simulink model "RCAM_sim"  (R2023a)
settings: Solver=VariableStepAuto  StartTime=0.0  StopTime=t_sim  RelTol=1e-3
InitFcn:
  | % clc
  | % clear
  | % RCAM_init
  | % RCAM_init_trimmed
  | RCAM_constants
  | 
  | % Independent run (Untrimmed): Use lines 1,2,3,5
  | % Independent run (Trimmed): Use lines 1,2,4,5
  | % Trimming: Use line 5 only
values from neighbouring files (symbols this model uses):
  a0 = 15.212    [RCAM0_model.m]    (also in RCAM_constants.m; RCAM_constants.mat)
  a1 = -155.2    [RCAM0_model.m]    (also in RCAM_constants.m; RCAM_constants.mat)
  a2 = 609.2    [RCAM0_model.m]    (also in RCAM_constants.m; RCAM_constants.mat)
  a3 = -768.5    [RCAM0_model.m]    (also in RCAM_constants.m; RCAM_constants.mat)
  alpha_L0 = deg2rad(-11.5)    [RCAM0_model.m]    (also in RCAM_constants.m; RCAM_constants.mat = -0.200712863979)
  alpha_switch = deg2rad(14.5)    [RCAM0_model.m]    (also in RCAM_constants.m; RCAM_constants.mat = 0.253072741539)
  cbar = 6.6    [RCAM0_model.m]    (also in RCAM_constants.m; RCAM_constants.mat)
  cd_c1 = 0.654    [RCAM_constants.m]    (also in RCAM_constants.mat)
  cd_c2 = 0.13    [RCAM_constants.m]    (also in RCAM_constants.mat)
  cd_m1 = 5.5    [RCAM_constants.m]    (also in RCAM_constants.mat)
  cd_m2 = 0.07    [RCAM_constants.m]    (also in RCAM_constants.mat)
  dCYdbeta = -1.6    [RCAM_constants.m]    (also in RCAM_constants.mat)
  dCYdRud = 0.24    [RCAM_constants.m]    (also in RCAM_constants.mat)
  depsda = 0.25    [RCAM0_model.m]    (also in RCAM_constants.m; RCAM_constants.mat)
  dumax = deg2rad(dumax)    [RCAM_constants.m]    (also in RCAM_constants.mat = [1.0471975512 1.0471975512 1.0471975512 0.0349065850399 0.03)
  g = 9.81    [RCAM0_model.m]    (also in RCAM_constants.m; RCAM_constants.mat)
  lt = 24.8    [RCAM0_model.m]    (also in RCAM_constants.m; RCAM_constants.mat)
  m = 120000    [RCAM0_model.m]    (also in RCAM_constants.m; RCAM_constants.mat)
  n = 5.5    [RCAM0_model.m]    (also in RCAM_constants.m; RCAM_constants.mat)
  S = 260    [RCAM0_model.m]    (also in RCAM_constants.m; RCAM_constants.mat)
  St = 64    [RCAM0_model.m]    (also in RCAM_constants.m; RCAM_constants.mat)
  u0 = [0 ... (first row only)    [RCAM0_init.m]    (also in RCAM_constants.mat = [0 -0.194874130949 0 0.0795600512836 0.0795600512836]; RCAM_dynamics.m = u; RCAM_init.m = deg2rad(u0); RCAM_init2.m = ustar)
  umax = deg2rad(umax)    [RCAM0_model.m]    (also in RCAM_constants.m; RCAM_constants.mat = [0.436332312999 0.174532925199 0.523598775598 0.174532925199)
  umin = deg2rad(umin)    [RCAM0_model.m]    (also in RCAM_constants.m; RCAM_constants.mat = [-0.436332312999 -0.436332312999 -0.523598775598 0.008726646)
  Xac = 0.12*cbar    (= 0.792)    [RCAM0_model.m]    (also in RCAM_constants.m; RCAM_constants.mat)
  Xcg = 0.23*cbar    (= 1.518)    [RCAM0_model.m]    (also in RCAM_constants.m; RCAM_constants.mat)
  Yac = 0    [RCAM0_model.m]    (also in RCAM_constants.m; RCAM_constants.mat)
  Ycg = 0    [RCAM0_model.m]    (also in RCAM_constants.m; RCAM_constants.mat)
  Zac = 0    [RCAM0_model.m]    (also in RCAM_constants.m; RCAM_constants.mat)
  Zcg = 0.1*cbar    (= 0.66)    [RCAM0_model.m]    (also in RCAM_constants.m; RCAM_constants.mat)
libraries: simulink_extras x12, aerolibactuator x5, slpidlib x3, matrix_library x3, sharedutil x2, shared6dof x1, aerolibatmos2 x1
settings Model: Creator=Reggie Johanes  LastModifiedBy=Reggie Johanes

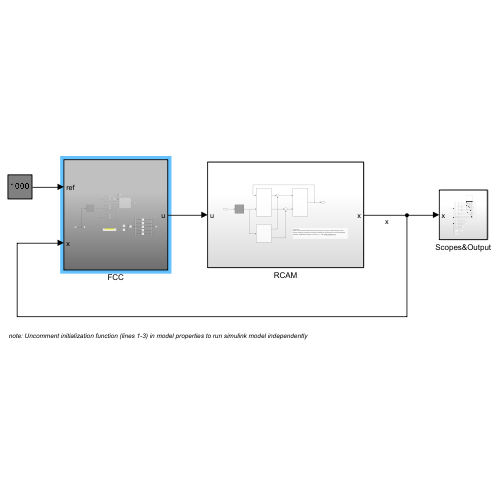
[thumbnail: Simulink's stored preview of the top-level diagram]
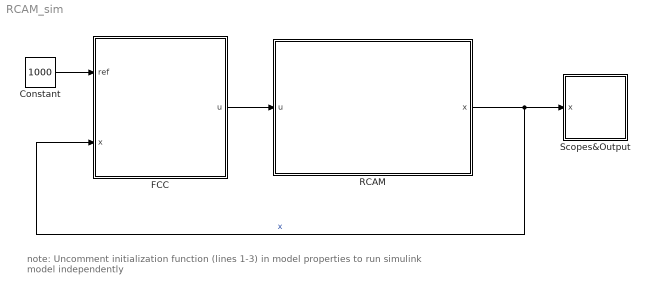
== system RCAM_sim ==
  note: note: Uncomment initialization function (lines 1-3) in model properties to run simulink model independently
  Constant : Constant  Value=1000
  FCC : Subsystem
  RCAM : Subsystem
  Scopes&Output : Subsystem
  wires:
  FCC/1(u) -> RCAM/1(u)
  RCAM/1(x) -> FCC/2(x), Scopes&Output/1(x)  "x"
  Constant/1 -> FCC/1(ref)

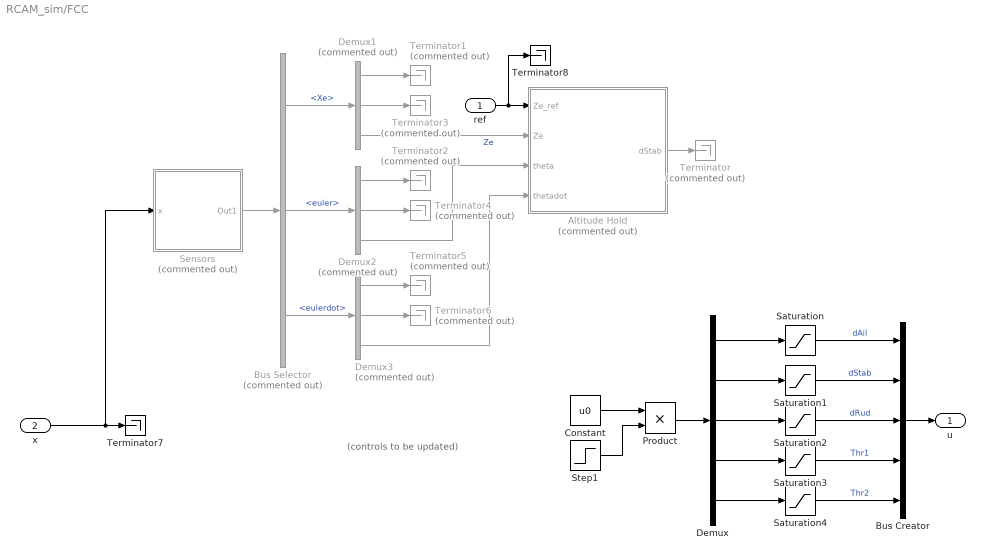
== system RCAM_sim/FCC ==
  note: (controls to be updated)
  ref : Inport
  x : Inport  Port=2
  Altitude Hold : Subsystem  Commented=on
  Bus Creator : BusCreator  Inputs=5
  Bus Selector : BusSelector  Commented=on  OutputSignals=Xe,euler,eulerdot
  Constant : Constant  Value=u0
  Demux : Demux  Outputs=5
  Demux1 : Demux  Commented=on  Outputs=3
  Demux2 : Demux  Commented=on  Outputs=3
  Demux3 : Demux  Commented=on  Outputs=3
  Product : Product
  Saturation : Saturate  UpperLimit=umax(1)  LowerLimit=umin(1)
  Saturation1 : Saturate  UpperLimit=umax(2)  LowerLimit=umin(2)
  Saturation2 : Saturate  UpperLimit=umax(3)  LowerLimit=umin(3)
  Saturation3 : Saturate  UpperLimit=umax(4)  LowerLimit=umin(4)
  Saturation4 : Saturate  UpperLimit=umax(5)  LowerLimit=umin(5)
  Sensors : Subsystem  Commented=on
  Step1 : Step  Time=0  SampleTime=0
  Terminator{,1..6} (7 alike) : Terminator  Commented=on
  Terminator7 : Terminator
  Terminator8 : Terminator
  u : Outport
  wires:
  ref/1 -> Terminator8/1, Altitude Hold/1(Ze_ref)
  x/1 -> Sensors/1(x), Terminator7/1
  Step1/1 -> Product/2
  Product/1 -> Demux/1
  Demux/5 -> Saturation4/1
  Demux/4 -> Saturation3/1
  Demux/3 -> Saturation2/1
  Demux/2 -> Saturation1/1
  Demux/1 -> Saturation/1
  Bus Creator/1 -> u/1
  Bus Selector/1 -> Demux1/1  "<Xe>"
  Bus Selector/2 -> Demux2/1  "<euler>"
  Saturation/1 -> Bus Creator/1  "dAil"
  Saturation1/1 -> Bus Creator/2  "dStab"
  Saturation2/1 -> Bus Creator/3  "dRud"
  Saturation3/1 -> Bus Creator/4  "Thr1"
  Saturation4/1 -> Bus Creator/5  "Thr2"
  Demux1/1 -> Terminator1/1
  Demux1/2 -> Terminator3/1
  Bus Selector/3 -> Demux3/1  "<eulerdot>"
  Demux1/3 -> Altitude Hold/2(Ze)  "Ze"
  Demux2/2 -> Terminator4/1
  Demux2/1 -> Terminator2/1
  Demux3/1 -> Terminator5/1
  Demux3/2 -> Terminator6/1
  Demux2/3 -> Altitude Hold/3(theta)
  Demux3/3 -> Altitude Hold/4(thetadot)
  Constant/1 -> Product/1
  Altitude Hold/1(dStab) -> Terminator/1
  Sensors/1(Out1) -> Bus Selector/1

== system RCAM_sim/RCAM ==
  note: Reference:
      | Group for Aeronautical Research and Technology in Europe, "Robust Flight Control Design Challenge Problem Formulation and Manual: the Research Civil Aircraft Model (RCAM)", GARTEUR/TP-0883. February 17, 1997 ( https://garteur.org )
  u : Inport
  Actuators : Subsystem
  Aerodynamics : Subsystem
  EOM&Environment : Subsystem
  Propulsion : Subsystem
  Sum : Sum  Inputs=|++
  Sum1 : Sum  Inputs=|++
  x : Outport
  wires:
  u/1 -> Actuators/1(In1)
  Aerodynamics/1(F_a) -> Sum/1
  Aerodynamics/2(M_a) -> Sum1/1
  Sum/1 -> EOM&Environment/1(F)
  Sum1/1 -> EOM&Environment/2(M)
  Propulsion/1(F_e) -> Sum/2
  Propulsion/2(M_e) -> Sum1/2
  EOM&Environment/1(x) -> Aerodynamics/1(x), x/1
  Actuators/1(Out1) -> Propulsion/1(u), Aerodynamics/2(u)

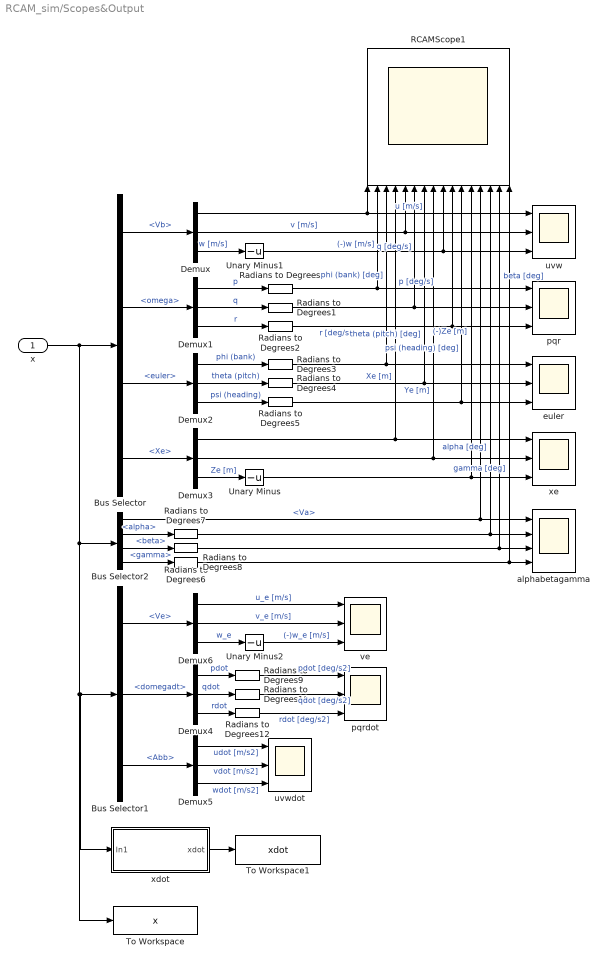
== system RCAM_sim/Scopes&Output ==
  x : Inport
  Bus Selector : BusSelector  OutputSignals=Vb,omega,euler,Xe
  Bus Selector1 : BusSelector  OutputSignals=Ve,domegadt,Abb
  Bus Selector2 : BusSelector  OutputSignals=Va,alpha,beta,gamma
  Demux{,1..6} (7 alike) : Demux  Outputs=3
  RCAMScope1 : Scope  NumInputPorts=16
  Radians to Degrees{,1..10,12} (12 alike) : simulink_extras/Transformations/Radians to Degrees
  To Workspace : ToWorkspace  VariableName=x  SaveFormat=Timeseries  SampleTime=-1
  To Workspace1 : ToWorkspace  VariableName=xdot  SampleTime=-1
  Unary Minus : UnaryMinus
  Unary Minus1 : UnaryMinus
  Unary Minus2 : UnaryMinus
  alphabetagamma : Scope  NumInputPorts=4
  euler : Scope  NumInputPorts=3
  pqr : Scope  NumInputPorts=3
  pqrdot : Scope  NumInputPorts=3
  uvw : Scope  NumInputPorts=3
  uvwdot : Scope  NumInputPorts=3
  ve : Scope  NumInputPorts=3
  xdot : Subsystem
  xe : Scope  NumInputPorts=3
  wires:
  x/1 -> To Workspace/1, xdot/1(In1), Bus Selector1/1, Bus Selector2/1, Bus Selector/1
  Bus Selector/1 -> Demux/1  "<Vb>"
  Bus Selector/2 -> Demux1/1  "<omega>"
  Bus Selector/3 -> Demux2/1  "<euler>"
  Demux/1 -> uvw/1, RCAMScope1/1  "u [m/s]"
  Demux1/2 -> Radians to Degrees1/1  "q"
  Demux/3 -> Unary Minus1/1  "w [m/s]"
  Demux/2 -> uvw/2, RCAMScope1/5  "v [m/s]"
  Demux1/1 -> Radians to Degrees/1  "p"
  Demux1/3 -> Radians to Degrees2/1  "r"
  Demux2/2 -> Radians to Degrees4/1  "theta (pitch)"
  Demux2/3 -> Radians to Degrees5/1  "psi (heading)"
  Bus Selector/4 -> Demux3/1  "<Xe>"
  Demux3/1 -> xe/1, RCAMScope1/4  "Xe [m]"
  Demux3/2 -> xe/2, RCAMScope1/8  "Ye [m]"
  Demux3/3 -> Unary Minus/1  "Ze [m]"
  Demux2/1 -> Radians to Degrees3/1  "phi (bank)"
  Demux4/3 -> Radians to Degrees12/1  "rdot"
  Demux4/2 -> Radians to Degrees10/1  "qdot"
  Bus Selector1/2 -> Demux4/1  "<domegadt>"
  Demux4/1 -> Radians to Degrees9/1  "pdot"
  Demux5/1 -> uvwdot/1  "udot [m/s2]"
  Bus Selector1/3 -> Demux5/1  "<Abb>"
  Demux5/2 -> uvwdot/2  "vdot [m/s2]"
  Demux5/3 -> uvwdot/3  "wdot [m/s2]"
  Radians to Degrees/1 -> pqr/1, RCAMScope1/2  "p [deg/s]"
  Radians to Degrees1/1 -> pqr/2, RCAMScope1/6  "q [deg/s]"
  Radians to Degrees2/1 -> pqr/3, RCAMScope1/10  "r [deg/s]"
  Radians to Degrees3/1 -> euler/1, RCAMScope1/3  "phi (bank) [deg]"
  Radians to Degrees4/1 -> euler/2, RCAMScope1/7  "theta (pitch) [deg]"
  Radians to Degrees5/1 -> euler/3, RCAMScope1/11  "psi (heading) [deg]"
  Unary Minus/1 -> xe/3, RCAMScope1/12  "(-)Ze [m]"
  Bus Selector2/3 -> Radians to Degrees6/1  "<beta>"
  Bus Selector2/1 -> RCAMScope1/13, alphabetagamma/1  "<Va>"
  Bus Selector2/2 -> Radians to Degrees7/1  "<alpha>"
  Radians to Degrees6/1 -> RCAMScope1/15, alphabetagamma/3  "beta [deg]"
  Radians to Degrees7/1 -> RCAMScope1/14, alphabetagamma/2  "alpha [deg]"
  Demux6/3 -> Unary Minus2/1  "w_e"
  Demux6/2 -> ve/2  "v_e [m/s]"
  Bus Selector1/1 -> Demux6/1  "<Ve>"
  Demux6/1 -> ve/1  "u_e [m/s]"
  Unary Minus2/1 -> ve/3  "(-)w_e [m/s]"
  Unary Minus1/1 -> uvw/3, RCAMScope1/9  "(-)w [m/s]"
  Bus Selector2/4 -> Radians to Degrees8/1  "<gamma>"
  Radians to Degrees8/1 -> RCAMScope1/16, alphabetagamma/4  "gamma [deg]"
  Radians to Degrees9/1 -> pqrdot/1  "pdot [deg/s2]"
  Radians to Degrees10/1 -> pqrdot/2  "qdot [deg/s2]"
  Radians to Degrees12/1 -> pqrdot/3  "rdot [deg/s2]"
  xdot/1(xdot) -> To Workspace1/1

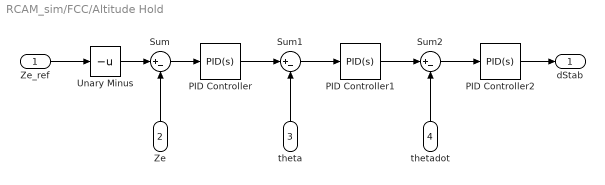
== system RCAM_sim/FCC/Altitude Hold ==
  Ze_ref : Inport
  Ze : Inport  Port=2
  theta : Inport  Port=3
  thetadot : Inport  Port=4
  PID Controller : slpidlib/PID Controller  Controller=PID  Form=Parallel  TimeDomain=Continuous-time  UseExternalTs=off  SampleTime=-1  IntegratorMethod=Forward Euler  FilterMethod=Forward Euler  ControllerParametersSource=internal  P=-2.5  I=0  UseKiTs=off  D=0  N=100  UseFilter=on  TunerSelectOption=Transfer Function Based (PID Tuner App)  InitialConditionSource=internal  InitialConditionForIntegrator=0  InitialConditionForFilter=0  DifferentiatorICPrevScaledInput=0  ExternalReset=none  TrackingMode=off  Kt=1  LimitOutput=off  SatLimitsSource=internal  UpperSaturationLimit=inf  LowerSaturationLimit=-inf  LinearizeAsGain=on  AntiWindupMode=none  Kb=1  LimitIntegrator=off  UpperIntegratorSaturationLimit=inf  LowerIntegratorSaturationLimit=-inf  POutMin=[]  POutMax=[]  IOutMin=[]  IOutMax=[]  DOutMin=[]  DOutMax=[]  NOutMin=[]  NOutMax=[]  SumOutMin=[]  SumOutMax=[]  SaturationOutMin=[]  SaturationOutMax=[]  PParamMin=[]  PParamMax=[]  IParamMin=[]  IParamMax=[]  DParamMin=[]  DParamMax=[]  NParamMin=[]  NParamMax=[]  KbParamMin=[]  KbParamMax=[]  KtParamMin=[]  KtParamMax=[]  KbOutMin=[]  KbOutMax=[]  KtOutMin=[]  KtOutMax=[]  IntegratorOutMin=[]  IntegratorOutMax=[]  FilterOutMin=[]  FilterOutMax=[]  SumI1OutMin=[]  SumI1OutMax=[]  SumI2OutMin=[]  SumI2OutMax=[]  SumI3OutMin=[]  SumI3OutMax=[]  SumI4OutMin=[]  SumI4OutMax=[]  SumDOutMin=[]  SumDOutMax=[]  DifferentiatorOutMin=[]  DifferentiatorOutMax=[]  FilterDiffOutCoefMin=[]  FilterDiffOutCoefMax=[]  ReciprocalOutMin=[]  ReciprocalOutMax=[]  SumDenOutMin=[]  SumDenOutMax=[]  SumNumOutMin=[]  SumNumOutMax=[]  DivideOutMin=[]  DivideOutMax=[]  UdiffTsProdOutMin=[]  UdiffTsProdOutMax=[]  NTsProdOutMin=[]  NTsProdOutMax=[]  UintegralTsProdOutMin=[]  UintegralTsProdOutMax=[]  UngainTsProdOutMin=[]  UngainTsProdOutMax=[]  ClampingZeroOutDataTypeStr=Inherit: Inherit via back propagation  ClampingZeroOutMin=[]  ClampingZeroOutMax=[]  FilterDenConstantOutDataTypeStr=Inherit: Inherit via back propagation  FilterDenConstantOutMin=[]  FilterDenConstantOutMax=[]  PCopyOutDataTypeStr=Inherit: Inherit via back propagation  PCopyOutMin=[]  PCopyOutMax=[]  NCopyOutDataTypeStr=Inherit: Inherit via back propagation  NCopyOutMin=[]  NCopyOutMax=[]  IntegratorContinuousStateAttributes=''  IntegratorStateMustResolveToSignalObject=off  IntegratorRTWStateStorageClass=Auto  FilterContinuousStateAttributes=''  FilterStateMustResolveToSignalObject=off  FilterRTWStateStorageClass=Auto  ParallelPVariant=InternalParameters  IdealPVariant=Disabled  IVariant=InternalParameters  DVariant=InternalParameters  IntegratorVariant=Continuous  SatVariant=Disabled  AWVariant=Passthrough  PCopyVariant=Disabled  TRVariant=Disabled  FdbkBlocksVariant=Forward  IdealPFdbkVariant=Disabled  SatFdbkVariant=Disabled  DerivativeFilterVariant=ContFilter  NVariant=InternalParameters  NCopyVariant=Disabled  FilterICVariant=InternalICsFilter  IntegratorICVariant=InternalICs  ExternalResetVariant=Disabled  TRSumVariant=Passthrough  SumFdbkVariant=Disabled  SumVariant=Sum_PID  TsampFilterVariant=InternalTs  TsampNgainVariant=Passthrough  TsampIntegralVariant=Disabled_SignalSpec  ExternalSaturationOutDataTypeStr=Inherit: Same as second input
  PID Controller1 : slpidlib/PID Controller  Controller=PID  Form=Parallel  TimeDomain=Continuous-time  UseExternalTs=off  SampleTime=-1  IntegratorMethod=Forward Euler  FilterMethod=Forward Euler  ControllerParametersSource=internal  P=1.5  I=0  UseKiTs=off  D=0  N=100  UseFilter=on  TunerSelectOption=Transfer Function Based (PID Tuner App)  InitialConditionSource=internal  InitialConditionForIntegrator=0  InitialConditionForFilter=0  DifferentiatorICPrevScaledInput=0  ExternalReset=none  TrackingMode=off  Kt=1  LimitOutput=off  SatLimitsSource=internal  UpperSaturationLimit=inf  LowerSaturationLimit=-inf  LinearizeAsGain=on  AntiWindupMode=none  Kb=1  LimitIntegrator=off  UpperIntegratorSaturationLimit=inf  LowerIntegratorSaturationLimit=-inf  POutMin=[]  POutMax=[]  IOutMin=[]  IOutMax=[]  DOutMin=[]  DOutMax=[]  NOutMin=[]  NOutMax=[]  SumOutMin=[]  SumOutMax=[]  SaturationOutMin=[]  SaturationOutMax=[]  PParamMin=[]  PParamMax=[]  IParamMin=[]  IParamMax=[]  DParamMin=[]  DParamMax=[]  NParamMin=[]  NParamMax=[]  KbParamMin=[]  KbParamMax=[]  KtParamMin=[]  KtParamMax=[]  KbOutMin=[]  KbOutMax=[]  KtOutMin=[]  KtOutMax=[]  IntegratorOutMin=[]  IntegratorOutMax=[]  FilterOutMin=[]  FilterOutMax=[]  SumI1OutMin=[]  SumI1OutMax=[]  SumI2OutMin=[]  SumI2OutMax=[]  SumI3OutMin=[]  SumI3OutMax=[]  SumI4OutMin=[]  SumI4OutMax=[]  SumDOutMin=[]  SumDOutMax=[]  DifferentiatorOutMin=[]  DifferentiatorOutMax=[]  FilterDiffOutCoefMin=[]  FilterDiffOutCoefMax=[]  ReciprocalOutMin=[]  ReciprocalOutMax=[]  SumDenOutMin=[]  SumDenOutMax=[]  SumNumOutMin=[]  SumNumOutMax=[]  DivideOutMin=[]  DivideOutMax=[]  UdiffTsProdOutMin=[]  UdiffTsProdOutMax=[]  NTsProdOutMin=[]  NTsProdOutMax=[]  UintegralTsProdOutMin=[]  UintegralTsProdOutMax=[]  UngainTsProdOutMin=[]  UngainTsProdOutMax=[]  ClampingZeroOutDataTypeStr=Inherit: Inherit via back propagation  ClampingZeroOutMin=[]  ClampingZeroOutMax=[]  FilterDenConstantOutDataTypeStr=Inherit: Inherit via back propagation  FilterDenConstantOutMin=[]  FilterDenConstantOutMax=[]  PCopyOutDataTypeStr=Inherit: Inherit via back propagation  PCopyOutMin=[]  PCopyOutMax=[]  NCopyOutDataTypeStr=Inherit: Inherit via back propagation  NCopyOutMin=[]  NCopyOutMax=[]  IntegratorContinuousStateAttributes=''  IntegratorStateMustResolveToSignalObject=off  IntegratorRTWStateStorageClass=Auto  FilterContinuousStateAttributes=''  FilterStateMustResolveToSignalObject=off  FilterRTWStateStorageClass=Auto  ParallelPVariant=InternalParameters  IdealPVariant=Disabled  IVariant=InternalParameters  DVariant=InternalParameters  IntegratorVariant=Continuous  SatVariant=Disabled  AWVariant=Passthrough  PCopyVariant=Disabled  TRVariant=Disabled  FdbkBlocksVariant=Forward  IdealPFdbkVariant=Disabled  SatFdbkVariant=Disabled  DerivativeFilterVariant=ContFilter  NVariant=InternalParameters  NCopyVariant=Disabled  FilterICVariant=InternalICsFilter  IntegratorICVariant=InternalICs  ExternalResetVariant=Disabled  TRSumVariant=Passthrough  SumFdbkVariant=Disabled  SumVariant=Sum_PID  TsampFilterVariant=InternalTs  TsampNgainVariant=Passthrough  TsampIntegralVariant=Disabled_SignalSpec  ExternalSaturationOutDataTypeStr=Inherit: Same as second input
  PID Controller2 : slpidlib/PID Controller  Controller=PID  Form=Parallel  TimeDomain=Continuous-time  UseExternalTs=off  SampleTime=-1  IntegratorMethod=Forward Euler  FilterMethod=Forward Euler  ControllerParametersSource=internal  P=-2.5  I=0  UseKiTs=off  D=0  N=100  UseFilter=on  TunerSelectOption=Transfer Function Based (PID Tuner App)  InitialConditionSource=internal  InitialConditionForIntegrator=0  InitialConditionForFilter=0  DifferentiatorICPrevScaledInput=0  ExternalReset=none  TrackingMode=off  Kt=1  LimitOutput=off  SatLimitsSource=internal  UpperSaturationLimit=inf  LowerSaturationLimit=-inf  LinearizeAsGain=on  AntiWindupMode=none  Kb=1  LimitIntegrator=off  UpperIntegratorSaturationLimit=inf  LowerIntegratorSaturationLimit=-inf  POutMin=[]  POutMax=[]  IOutMin=[]  IOutMax=[]  DOutMin=[]  DOutMax=[]  NOutMin=[]  NOutMax=[]  SumOutMin=[]  SumOutMax=[]  SaturationOutMin=[]  SaturationOutMax=[]  PParamMin=[]  PParamMax=[]  IParamMin=[]  IParamMax=[]  DParamMin=[]  DParamMax=[]  NParamMin=[]  NParamMax=[]  KbParamMin=[]  KbParamMax=[]  KtParamMin=[]  KtParamMax=[]  KbOutMin=[]  KbOutMax=[]  KtOutMin=[]  KtOutMax=[]  IntegratorOutMin=[]  IntegratorOutMax=[]  FilterOutMin=[]  FilterOutMax=[]  SumI1OutMin=[]  SumI1OutMax=[]  SumI2OutMin=[]  SumI2OutMax=[]  SumI3OutMin=[]  SumI3OutMax=[]  SumI4OutMin=[]  SumI4OutMax=[]  SumDOutMin=[]  SumDOutMax=[]  DifferentiatorOutMin=[]  DifferentiatorOutMax=[]  FilterDiffOutCoefMin=[]  FilterDiffOutCoefMax=[]  ReciprocalOutMin=[]  ReciprocalOutMax=[]  SumDenOutMin=[]  SumDenOutMax=[]  SumNumOutMin=[]  SumNumOutMax=[]  DivideOutMin=[]  DivideOutMax=[]  UdiffTsProdOutMin=[]  UdiffTsProdOutMax=[]  NTsProdOutMin=[]  NTsProdOutMax=[]  UintegralTsProdOutMin=[]  UintegralTsProdOutMax=[]  UngainTsProdOutMin=[]  UngainTsProdOutMax=[]  ClampingZeroOutDataTypeStr=Inherit: Inherit via back propagation  ClampingZeroOutMin=[]  ClampingZeroOutMax=[]  FilterDenConstantOutDataTypeStr=Inherit: Inherit via back propagation  FilterDenConstantOutMin=[]  FilterDenConstantOutMax=[]  PCopyOutDataTypeStr=Inherit: Inherit via back propagation  PCopyOutMin=[]  PCopyOutMax=[]  NCopyOutDataTypeStr=Inherit: Inherit via back propagation  NCopyOutMin=[]  NCopyOutMax=[]  IntegratorContinuousStateAttributes=''  IntegratorStateMustResolveToSignalObject=off  IntegratorRTWStateStorageClass=Auto  FilterContinuousStateAttributes=''  FilterStateMustResolveToSignalObject=off  FilterRTWStateStorageClass=Auto  ParallelPVariant=InternalParameters  IdealPVariant=Disabled  IVariant=InternalParameters  DVariant=InternalParameters  IntegratorVariant=Continuous  SatVariant=Disabled  AWVariant=Passthrough  PCopyVariant=Disabled  TRVariant=Disabled  FdbkBlocksVariant=Forward  IdealPFdbkVariant=Disabled  SatFdbkVariant=Disabled  DerivativeFilterVariant=ContFilter  NVariant=InternalParameters  NCopyVariant=Disabled  FilterICVariant=InternalICsFilter  IntegratorICVariant=InternalICs  ExternalResetVariant=Disabled  TRSumVariant=Passthrough  SumFdbkVariant=Disabled  SumVariant=Sum_PID  TsampFilterVariant=InternalTs  TsampNgainVariant=Passthrough  TsampIntegralVariant=Disabled_SignalSpec  ExternalSaturationOutDataTypeStr=Inherit: Same as second input
  Sum : Sum  Inputs=|+-
  Sum1 : Sum  Inputs=|+-
  Sum2 : Sum  Inputs=|+-
  Unary Minus : UnaryMinus
  dStab : Outport
  wires:
  Ze_ref/1 -> Unary Minus/1
  Unary Minus/1 -> Sum/1
  Ze/1 -> Sum/2
  Sum/1 -> PID Controller/1
  Sum1/1 -> PID Controller1/1
  Sum2/1 -> PID Controller2/1
  PID Controller/1 -> Sum1/1
  theta/1 -> Sum1/2
  PID Controller1/1 -> Sum2/1
  thetadot/1 -> Sum2/2
  PID Controller2/1 -> dStab/1

== system RCAM_sim/FCC/Sensors ==
  x : Inport
  Out1 : Outport
  wires:
  x/1 -> Out1/1

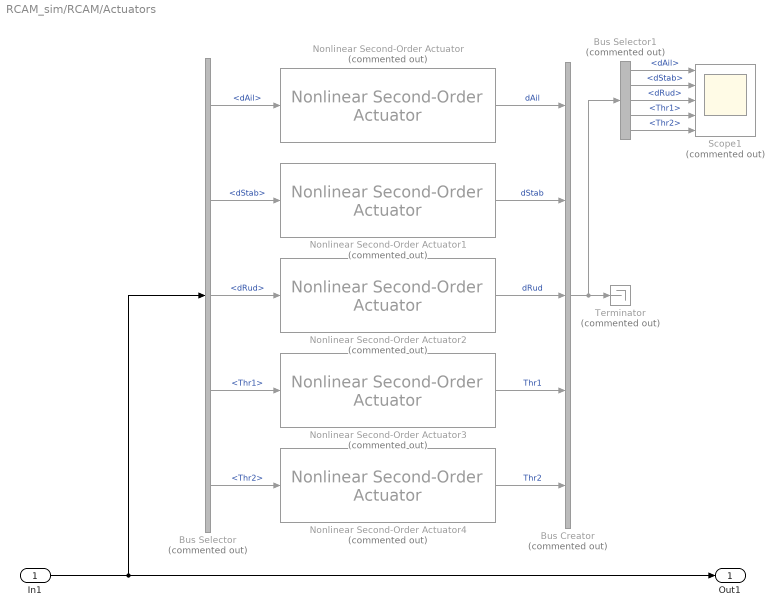
== system RCAM_sim/RCAM/Actuators ==
  In1 : Inport
  Bus Creator : BusCreator  Commented=on  Inputs=5
  Bus Selector : BusSelector  Commented=on  OutputSignals=dAil,dStab,dRud,Thr1,Thr2
  Bus Selector1 : BusSelector  Commented=on  OutputSignals=dAil,dStab,dRud,Thr1,Thr2
  Nonlinear Second-Order Actuator : aerolibactuator/Nonlinear Second-Order Actuator  Commented=on  wn_fin=1  z_fin=0.3  fin_max=umax(1)  fin_min=umin(1)  fin_maxrate=dumax(1)  fin_act_0=u0(1)  fin_act_vel=0
  Nonlinear Second-Order Actuator1 : aerolibactuator/Nonlinear Second-Order Actuator  Commented=on  wn_fin=1  z_fin=0.3  fin_max=umax(2)  fin_min=umin(2)  fin_maxrate=dumax(2)  fin_act_0=u0(2)  fin_act_vel=0
  Nonlinear Second-Order Actuator2 : aerolibactuator/Nonlinear Second-Order Actuator  Commented=on  wn_fin=1  z_fin=0.3  fin_max=umax(3)  fin_min=umin(3)  fin_maxrate=dumax(3)  fin_act_0=u0(3)  fin_act_vel=0
  Nonlinear Second-Order Actuator3 : aerolibactuator/Nonlinear Second-Order Actuator  Commented=on  wn_fin=1  z_fin=0.3  fin_max=umax(4)  fin_min=umin(4)  fin_maxrate=dumax(4)  fin_act_0=u0(4)  fin_act_vel=0
  Nonlinear Second-Order Actuator4 : aerolibactuator/Nonlinear Second-Order Actuator  Commented=on  wn_fin=1  z_fin=0.3  fin_max=umax(5)  fin_min=umin(5)  fin_maxrate=dumax(5)  fin_act_0=u0(5)  fin_act_vel=0
  Scope1 : Scope  Commented=on  NumInputPorts=5
  Terminator : Terminator  Commented=on
  Out1 : Outport
  wires:
  In1/1 -> Bus Selector/1, Out1/1
  Nonlinear Second-Order Actuator/1 -> Bus Creator/1  "dAil"
  Nonlinear Second-Order Actuator1/1 -> Bus Creator/2  "dStab"
  Nonlinear Second-Order Actuator2/1 -> Bus Creator/3  "dRud"
  Nonlinear Second-Order Actuator3/1 -> Bus Creator/4  "Thr1"
  Nonlinear Second-Order Actuator4/1 -> Bus Creator/5  "Thr2"
  Bus Creator/1 -> Bus Selector1/1, Terminator/1
  Bus Selector/1 -> Nonlinear Second-Order Actuator/1  "<dAil>"
  Bus Selector/2 -> Nonlinear Second-Order Actuator1/1  "<dStab>"
  Bus Selector/3 -> Nonlinear Second-Order Actuator2/1  "<dRud>"
  Bus Selector/4 -> Nonlinear Second-Order Actuator3/1  "<Thr1>"
  Bus Selector/5 -> Nonlinear Second-Order Actuator4/1  "<Thr2>"
  Bus Selector1/5 -> Scope1/5  "<Thr2>"
  Bus Selector1/3 -> Scope1/3  "<dRud>"
  Bus Selector1/2 -> Scope1/2  "<dStab>"
  Bus Selector1/1 -> Scope1/1  "<dAil>"
  Bus Selector1/4 -> Scope1/4  "<Thr1>"

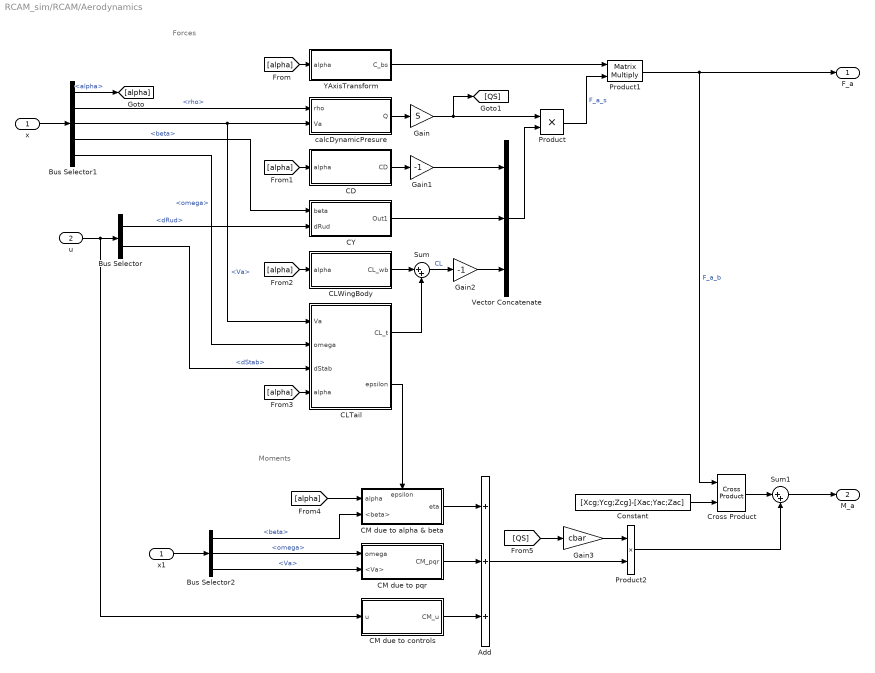
== system RCAM_sim/RCAM/Aerodynamics ==
  note: Moments
  note: Forces
  x : Inport
  u : Inport  Port=2
  Add : Sum  Inputs=+++
  Bus Selector : BusSelector  OutputSignals=dRud,dStab
  Bus Selector1 : BusSelector  OutputSignals=alpha,rho,Va,beta,omega
  Bus Selector2 : BusSelector  OutputSignals=beta,omega,Va
  CD : Subsystem
  CLTail : Subsystem
  CLWingBody : Subsystem
  CM due to alpha & beta : Subsystem
      settings: PortSchema="{\"entries\":[{\"content\":{\"sides\":[{\"content\":{\"connectorIds\":[\"In1\",\"In2\"]},\"type\":\"ConnectorPlacement.EquallySpacedRectSide\",\"uuid\":\"4ea81cfb-212a-42b7-a834-1cb32459f0c1\"},{\"content\":{\"connectorIds\":[\"Out1\"],\"side\":\"RIGHT\"},\"type\":\"ConnectorPlacement.EquallySpacedRectSide\",\"uuid\":\"0fcdfd01-09f5-4fd3-8241-6b6628318893\"},{\"content\":{\"connectorIds\":[\"In3\"],\"side\":\"TOP\"},\"type\":\"ConnectorPlacement.EquallySpacedRectSide\",\"uuid\":\"b9e9cc8b-be04-4675-a5d2-f8c3765db461\"}]},\"type\":\"ConnectorPlacement.EquallySpacedConnector\",\"uuid\":\"0a2dab64-2ac3-4f93-98ea-dd9c0c5e22da\"}],\"packageUris\":[\"http://schema.mathworks.com/mf0/Connector/R2020b\"],\"version\":\"1.0\"}"
  CM due to controls : Subsystem
  CM due to pqr : Subsystem
  CY : Subsystem
  Constant : Constant  Value=[Xcg;Ycg;Zcg]-[Xac;Yac;Zac]
  Cross Product : matrix_library/Cross Product
  Gain : Gain  Gain=S
  Gain1 : Gain  Gain=-1
  Gain2 : Gain  Gain=-1
  Gain3 : Gain  Gain=cbar
  Product : Product
  Product1 : Product  Multiplication=Matrix(*)
  Product2 : Product
  Sum : Sum  Inputs=|++
  Sum1 : Sum  Inputs=|++
  Vector Concatenate : Concatenate  NumInputs=3
  YAxisTransform : Subsystem
  calcDynamicPresure : Subsystem
  x1 : InportShadow
  F_a : Outport
  M_a : Outport  Port=2
  wires:
  x/1 -> Bus Selector1/1
  u/1 -> Bus Selector/1, CM due to controls/1(u)
  CLWingBody/1(CL_wb) -> Sum/1
  CLTail/1(CL_t) -> Sum/2
  Sum/1 -> Gain2/1  "CL"
  Bus Selector1/5 -> CLTail/2(omega)  "<omega>"
  Bus Selector1/2 -> calcDynamicPresure/1(rho)  "<rho>"
  Bus Selector1/3 -> CLTail/1(Va), calcDynamicPresure/2(Va)  "<Va>"
  Bus Selector1/4 -> CY/1(beta)  "<beta>"
  Bus Selector/2 -> CLTail/3(dStab)  "<dStab>"
  Bus Selector/1 -> CY/2(dRud)  "<dRud>"
  calcDynamicPresure/1(Q) -> Gain/1
  CD/1(CD) -> Gain1/1
  Gain1/1 -> Vector Concatenate/1
  CY/1(Out1) -> Vector Concatenate/2
  Gain2/1 -> Vector Concatenate/3
  Gain/1 -> [QS], Product/1
  Vector Concatenate/1 -> Product/2
  Product/1 -> Product1/2  "F_a_s"
  YAxisTransform/1(C_bs) -> Product1/1
  Product1/1 -> F_a/1, Cross Product/1  "F_a_b"
  CLTail/2(epsilon) -> CM due to alpha & beta/3(epsilon)
  Bus Selector1/1 -> [alpha]  "<alpha>"
  [alpha] -> YAxisTransform/1(alpha)
  [alpha] -> CD/1(alpha)
  [alpha] -> CLWingBody/1(alpha)
  [alpha] -> CLTail/4(alpha)
  [alpha] -> CM due to alpha & beta/1(alpha)
  CM due to alpha & beta/1(eta) -> Add/1
  CM due to pqr/1(CM_pqr) -> Add/2
  CM due to controls/1(CM_u) -> Add/3
  [QS] -> Gain3/1
  Gain3/1 -> Product2/1
  Add/1 -> Product2/2
  x1/1 -> Bus Selector2/1
  Bus Selector2/1 -> CM due to alpha & beta/2(<beta>)  "<beta>"
  Bus Selector2/2 -> CM due to pqr/1(omega)  "<omega>"
  Bus Selector2/3 -> CM due to pqr/2(<Va>)  "<Va>"
  Constant/1 -> Cross Product/2
  Cross Product/1 -> Sum1/1
  Product2/1 -> Sum1/2
  Sum1/1 -> M_a/1

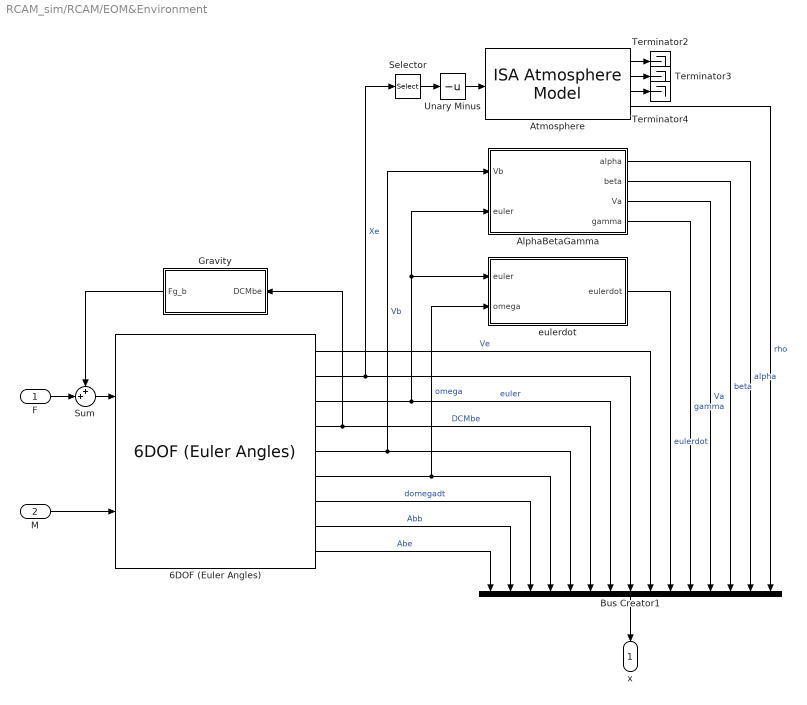
== system RCAM_sim/RCAM/EOM&Environment ==
  F : Inport
  M : Inport  Port=2
  6DOF (Euler Angles) : shared6dof/6DOF (Euler Angles)  units=Metric (MKS)  mtype=Fixed  rep=Euler Angles  xme_0=Xe0  Vm_0=Vb0  eul_0=euler0  pm_0=pqr0  mass_0=m  mass_e=0.5  mass_f=2.0  inertia=Ib  inertia_e=eye(3)  inertia_f=2*eye(3)  k_quat=1.0  vre_flag=on  abi_flag=on  aMode=0  xme_statename=''  Vm_statename=''  eul_statename=''  quat_statename=''  pm_statename=''  mass_statename=''
  AlphaBetaGamma : Subsystem
  Atmosphere : aerolibatmos2/ISA Atmosphere Model  custom=off  g=9.80665  gamma=1.4  R=287.0531  L=0.0065  h_trop=11000  h_strat=20000  rho0=1.225  P0=101325  T0=288.15  h0=0
  Bus Creator1 : BusCreator  Inputs=15
  Gravity : Subsystem
  Selector : Selector  InputPortWidth=3  IndexOptions=Index vector (dialog)  Indices=[3]  OutputSizes=1
  Sum : Sum  Inputs=++|
  Terminator2 : Terminator
  Terminator3 : Terminator
  Terminator4 : Terminator
  Unary Minus : UnaryMinus
  eulerdot : Subsystem
  x : Outport
  wires:
  F/1 -> Sum/2
  M/1 -> 6DOF (Euler Angles)/2
  6DOF (Euler Angles)/2 -> Bus Creator1/8, Selector/1  "Xe"
  Atmosphere/1 -> Terminator2/1
  Atmosphere/2 -> Terminator3/1
  Bus Creator1/1 -> x/1
  6DOF (Euler Angles)/5 -> Bus Creator1/5, AlphaBetaGamma/1(Vb)  "Vb"
  Atmosphere/3 -> Terminator4/1
  AlphaBetaGamma/1(alpha) -> Bus Creator1/14  "alpha"
  AlphaBetaGamma/2(beta) -> Bus Creator1/13  "beta"
  Atmosphere/4 -> Bus Creator1/15  "rho"
  6DOF (Euler Angles)/1 -> Bus Creator1/9  "Ve"
  6DOF (Euler Angles)/3 -> Bus Creator1/7, AlphaBetaGamma/2(euler), eulerdot/1(euler)  "euler"
  6DOF (Euler Angles)/4 -> Bus Creator1/6, Gravity/1(DCMbe)  "DCMbe"
  6DOF (Euler Angles)/6 -> eulerdot/2(omega), Bus Creator1/4  "omega"
  6DOF (Euler Angles)/7 -> Bus Creator1/3  "domegadt"
  6DOF (Euler Angles)/8 -> Bus Creator1/2  "Abb"
  6DOF (Euler Angles)/9 -> Bus Creator1/1  "Abe"
  AlphaBetaGamma/3(Va) -> Bus Creator1/12  "Va"
  Gravity/1(Fg_b) -> Sum/1
  Sum/1 -> 6DOF (Euler Angles)/1
  Selector/1 -> Unary Minus/1
  Unary Minus/1 -> Atmosphere/1
  AlphaBetaGamma/4(gamma) -> Bus Creator1/11  "gamma"
  eulerdot/1(eulerdot) -> Bus Creator1/10  "eulerdot"

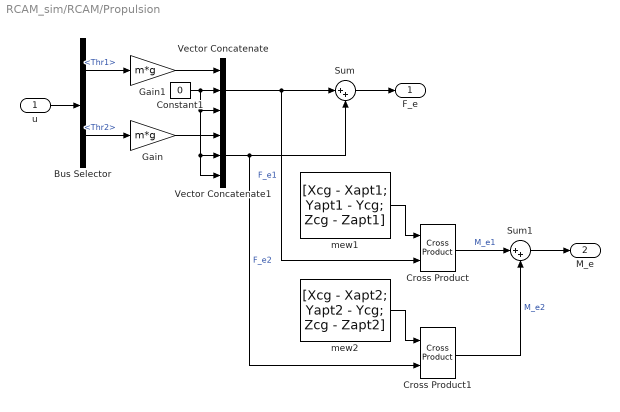
== system RCAM_sim/RCAM/Propulsion ==
  u : Inport
  Bus Selector : BusSelector  OutputSignals=Thr1,Thr2
  Constant1 : Constant  Value=0
  Cross Product : matrix_library/Cross Product
  Cross Product1 : matrix_library/Cross Product
  Gain : Gain  Gain=m*g
  Gain1 : Gain  Gain=m*g
  Sum : Sum  Inputs=|++
  Sum1 : Sum  Inputs=|++
  Vector Concatenate : Concatenate  NumInputs=3
  Vector Concatenate1 : Concatenate  NumInputs=3
  mew1 : Constant  Value=|
      | [Xcg - Xapt1;
      |  Yapt1 - Ycg;
      |   Zcg - Zapt1]
  mew2 : Constant  Value=|
      | [Xcg - Xapt2;
      |  Yapt2 - Ycg;
      |   Zcg - Zapt2]
  F_e : Outport
  M_e : Outport  Port=2
  wires:
  u/1 -> Bus Selector/1
  Bus Selector/1 -> Gain1/1  "<Thr1>"
  Bus Selector/2 -> Gain/1  "<Thr2>"
  Constant1/1 -> Vector Concatenate1/3, Vector Concatenate1/2, Vector Concatenate/3, Vector Concatenate/2
  Gain/1 -> Vector Concatenate1/1
  Vector Concatenate/1 -> Cross Product/2, Sum/1  "F_e1"
  Vector Concatenate1/1 -> Cross Product1/2, Sum/2  "F_e2"
  Sum/1 -> F_e/1
  mew1/1 -> Cross Product/1
  mew2/1 -> Cross Product1/1
  Cross Product/1 -> Sum1/1  "M_e1"
  Cross Product1/1 -> Sum1/2  "M_e2"
  Sum1/1 -> M_e/1
  Gain1/1 -> Vector Concatenate/1

== system RCAM_sim/Scopes&Output/xdot ==
  In1 : Inport
  Bus Selector3 : BusSelector  OutputSignals=Abb,domegadt,eulerdot,Ve
  Demux{,1..3} (4 alike) : Demux  Outputs=3
  Display : Display
  Vector Concatenate : Concatenate  NumInputs=12
  xdot : Outport
  wires:
  In1/1 -> Bus Selector3/1
  Bus Selector3/3 -> Demux3/1  "<eulerdot>"
  Bus Selector3/1 -> Demux/1  "<Abb>"
  Bus Selector3/2 -> Demux2/1  "<domegadt>"
  Bus Selector3/4 -> Demux1/1  "<Ve>"
  Vector Concatenate/1 -> Display/1, xdot/1
  Demux/1 -> Vector Concatenate/1  "udot"
  Demux/2 -> Vector Concatenate/2  "vdot"
  Demux/3 -> Vector Concatenate/3  "wdot"
  Demux2/1 -> Vector Concatenate/4  "pdot"
  Demux2/2 -> Vector Concatenate/5  "qdot"
  Demux2/3 -> Vector Concatenate/6  "qdot"
  Demux3/1 -> Vector Concatenate/7  "phidot"
  Demux3/2 -> Vector Concatenate/8  "thetadot"
  Demux3/3 -> Vector Concatenate/9  "psidot"
  Demux1/1 -> Vector Concatenate/10  "xedot"
  Demux1/2 -> Vector Concatenate/11  "yedot"
  Demux1/3 -> Vector Concatenate/12  "zedot"

== system RCAM_sim/RCAM/Aerodynamics/CD ==
  alpha : Inport
  Constant : Constant  Value=cd_c1
  Constant1 : Constant  Value=cd_c2
  Gain : Gain  Gain=cd_m1
  Gain1 : Gain  Gain=cd_m2
  Square : Math  Operator=square
  Sum : Sum  Inputs=|++
  Sum1 : Sum  Inputs=|++
  CD : Outport
  wires:
  alpha/1 -> Gain/1
  Constant/1 -> Sum/2
  Gain/1 -> Sum/1
  Sum/1 -> Square/1
  Square/1 -> Gain1/1
  Gain1/1 -> Sum1/1
  Constant1/1 -> Sum1/2
  Sum1/1 -> CD/1

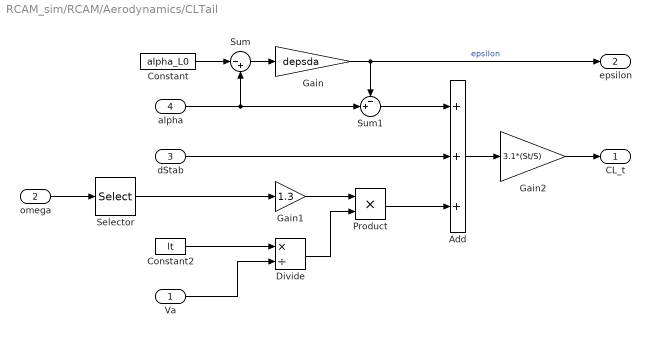
== system RCAM_sim/RCAM/Aerodynamics/CLTail ==
  Va : Inport
  omega : Inport  Port=2
  dStab : Inport  Port=3
  alpha : Inport  Port=4
  Add : Sum  Inputs=+++
  Constant : Constant  Value=alpha_L0
  Constant2 : Constant  Value=lt
  Divide : Product  Inputs=*/
  Gain : Gain  Gain=depsda
  Gain1 : Gain  Gain=1.3
  Gain2 : Gain  Gain=3.1*(St/S)
  Product : Product
  Selector : Selector  InputPortWidth=3  IndexOptions=Index vector (dialog)  Indices=[2]  OutputSizes=1
  Sum : Sum  Inputs=|-+
  Sum1 : Sum  Inputs=-+|
  CL_t : Outport
  epsilon : Outport  Port=2
  wires:
  alpha/1 -> Sum/2, Sum1/2
  Constant/1 -> Sum/1
  Sum/1 -> Gain/1
  Gain/1 -> epsilon/1, Sum1/1  "epsilon"
  Sum1/1 -> Add/1
  dStab/1 -> Add/2
  Va/1 -> Divide/2
  Constant2/1 -> Divide/1
  Gain1/1 -> Product/1
  Divide/1 -> Product/2
  Product/1 -> Add/3
  Add/1 -> Gain2/1
  Gain2/1 -> CL_t/1
  omega/1 -> Selector/1
  Selector/1 -> Gain1/1

== system RCAM_sim/RCAM/Aerodynamics/CLWingBody ==
  alpha : Inport
  Constant : Constant  Value=alpha_switch
  If : If  NumInputs=2  IfExpression=u1 >= u2
  If Action Subsystem : Subsystem  TreatAsAtomicUnit=on
  If Action Subsystem1 : Subsystem  TreatAsAtomicUnit=on
  Merge : Merge
  CL_wb : Outport
  wires:
  Constant/1 -> If/1
  alpha/1 -> If Action Subsystem/1(alpha), If Action Subsystem1/1(alpha), If/2
  If/2 -> If Action Subsystem/Action  "alpha>alpha_switch"
  If/1 -> If Action Subsystem1/Action  "alpha<=alpha_switch"
  If Action Subsystem1/1(CL_wb) -> Merge/1
  If Action Subsystem/1(Out1) -> Merge/2
  Merge/1 -> CL_wb/1

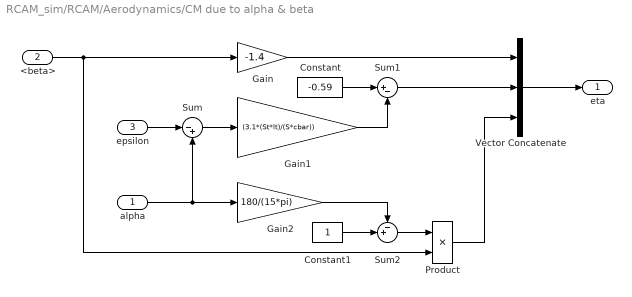
== system RCAM_sim/RCAM/Aerodynamics/CM due to alpha & beta ==
  alpha : Inport
  <beta> : Inport  Port=2
  epsilon : Inport  Port=3
  Constant : Constant  Value=-0.59
  Constant1 : Constant
  Gain : Gain  Gain=-1.4
  Gain1 : Gain  Gain=(3.1*(St*lt)/(S*cbar))
  Gain2 : Gain  Gain=180/(15*pi)
  Product : Product
  Sum : Sum  Inputs=|-+
  Sum1 : Sum  Inputs=|+-
  Sum2 : Sum  Inputs=-+|
  Vector Concatenate : Concatenate  NumInputs=3
  eta : Outport
  wires:
  <beta>/1 -> Product/2, Gain/1
  Gain/1 -> Vector Concatenate/1
  Vector Concatenate/1 -> eta/1
  alpha/1 -> Sum/2, Gain2/1
  epsilon/1 -> Sum/1
  Sum/1 -> Gain1/1
  Constant/1 -> Sum1/1
  Gain1/1 -> Sum1/2
  Sum1/1 -> Vector Concatenate/2
  Constant1/1 -> Sum2/2
  Gain2/1 -> Sum2/1
  Sum2/1 -> Product/1
  Product/1 -> Vector Concatenate/3

== system RCAM_sim/RCAM/Aerodynamics/CM due to controls ==
  u : Inport
  Bus Selector : BusSelector  OutputSignals=dAil,dStab,dRud
  Control Effectiveness Matrix : Constant  Value=|
      | [-0.6    0                           0.22;
      | 0    (-3.1*(St*lt)/(S*cbar))   0;
      |       0     0                         -0.63]
  Product : Product  Multiplication=Matrix(*)
  Vector Concatenate : Concatenate  NumInputs=3
  CM_u : Outport
  wires:
  Control Effectiveness Matrix/1 -> Product/1
  u/1 -> Bus Selector/1
  Bus Selector/1 -> Vector Concatenate/1  "<dAil>"
  Bus Selector/2 -> Vector Concatenate/2  "<dStab>"
  Bus Selector/3 -> Vector Concatenate/3  "<dRud>"
  Vector Concatenate/1 -> Product/2
  Product/1 -> CM_u/1

== system RCAM_sim/RCAM/Aerodynamics/CM due to pqr ==
  omega : Inport
  <Va> : Inport  Port=2
  Constant : Constant  Value=cbar
  Constant1 : Constant  Value=|
      | [-11   0                                5;
      |   0    (-4.03*(St*lt^2)/(S*cbar^2))  0;
      |   1.7   0                            -11.5]
  Divide : Product  Inputs=*/
  Product : Product
  Product1 : Product  Multiplication=Matrix(*)
  CM_pqr : Outport
  wires:
  Constant/1 -> Divide/1
  <Va>/1 -> Divide/2
  Divide/1 -> Product/1
  Constant1/1 -> Product/2
  Product/1 -> Product1/1
  omega/1 -> Product1/2
  Product1/1 -> CM_pqr/1

== system RCAM_sim/RCAM/Aerodynamics/CY ==
  beta : Inport
  dRud : Inport  Port=2
  Gain : Gain  Gain=dCYdbeta
  Gain1 : Gain  Gain=dCYdRud
  Sum : Sum  Inputs=|++
  Out1 : Outport
  wires:
  beta/1 -> Gain/1
  dRud/1 -> Gain1/1
  Gain/1 -> Sum/1
  Gain1/1 -> Sum/2
  Sum/1 -> Out1/1

== system RCAM_sim/RCAM/Aerodynamics/YAxisTransform ==
  alpha : Inport
  Constant : Constant  Value=0
  Constant1 : Constant
  Cos : Trigonometry  Operator=cos
  Create 3x3 Matrix : sharedutil/Create 3x3 Matrix  aMode=aMode
      settings: LibrarySourceBlock=aerolibutil/Create 3x3 Matrix
  Gain : Gain  Gain=-1
  Sin : Trigonometry
  C_bs : Outport
  wires:
  alpha/1 -> Sin/1, Cos/1
  Sin/1 -> Gain/1, Create 3x3 Matrix/7
  Cos/1 -> Create 3x3 Matrix/9, Create 3x3 Matrix/1
  Constant/1 -> Create 3x3 Matrix/8, Create 3x3 Matrix/6, Create 3x3 Matrix/4, Create 3x3 Matrix/2
  Gain/1 -> Create 3x3 Matrix/3
  Constant1/1 -> Create 3x3 Matrix/5
  Create 3x3 Matrix/1 -> C_bs/1

== system RCAM_sim/RCAM/Aerodynamics/calcDynamicPresure ==
  rho : Inport
  Va : Inport  Port=2
  Gain : Gain  Gain=0.5
  Product : Product
  Square : Math  Operator=square
  Q : Outport
  wires:
  Va/1 -> Square/1
  Square/1 -> Product/1
  rho/1 -> Gain/1
  Gain/1 -> Product/2
  Product/1 -> Q/1

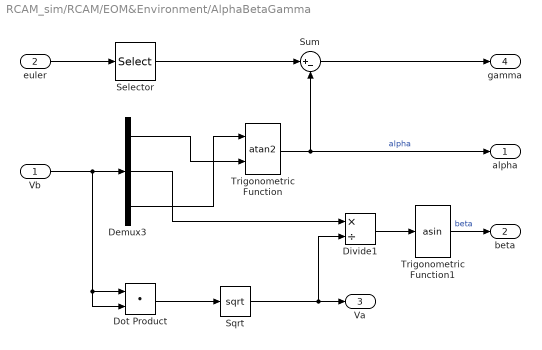
== system RCAM_sim/RCAM/EOM&Environment/AlphaBetaGamma ==
  Vb : Inport
  euler : Inport  Port=2
  Demux3 : Demux  Outputs=3
  Divide1 : Product  Inputs=*/
  Dot Product : DotProduct  OutDataTypeStr=Inherit: Inherit via internal rule
  Selector : Selector  InputPortWidth=3  IndexOptions=Index vector (dialog)  Indices=[2]  OutputSizes=1
  Sqrt : Sqrt
  Sum : Sum  Inputs=|+-
  Trigonometric Function : Trigonometry  Operator=atan2
  Trigonometric Function1 : Trigonometry  Operator=asin
  alpha : Outport
  beta : Outport  Port=2
  Va : Outport  Port=3
  gamma : Outport  Port=4
  wires:
  Vb/1 -> Dot Product/1, Dot Product/2, Demux3/1
  Trigonometric Function/1 -> alpha/1, Sum/2  "alpha"
  Demux3/2 -> Divide1/1
  Dot Product/1 -> Sqrt/1
  Demux3/3 -> Trigonometric Function/1
  Demux3/1 -> Trigonometric Function/2
  Divide1/1 -> Trigonometric Function1/1
  Sqrt/1 -> Divide1/2, Va/1
  Trigonometric Function1/1 -> beta/1  "beta"
  euler/1 -> Selector/1
  Selector/1 -> Sum/1
  Sum/1 -> gamma/1

== system RCAM_sim/RCAM/EOM&Environment/Gravity ==
  DCMbe : Inport
  Constant1 : Constant  Value=m*g
  Constant3 : Constant  Value=0
  Product3 : Product  Multiplication=Matrix(*)
  Vector Concatenate1 : Concatenate  NumInputs=3
  Fg_b : Outport
  wires:
  DCMbe/1 -> Product3/1
  Constant1/1 -> Vector Concatenate1/3
  Constant3/1 -> Vector Concatenate1/2, Vector Concatenate1/1
  Vector Concatenate1/1 -> Product3/2
  Product3/1 -> Fg_b/1  "F"

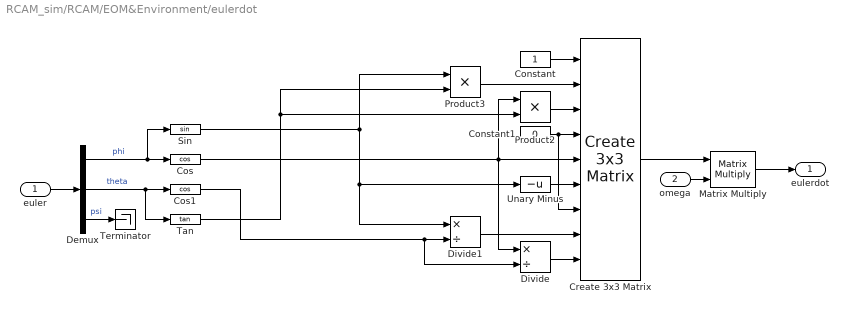
== system RCAM_sim/RCAM/EOM&Environment/eulerdot ==
  euler : Inport
  omega : Inport  Port=2
  Constant : Constant
  Constant1 : Constant  Value=0
  Cos : Trigonometry  Operator=cos
  Cos1 : Trigonometry  Operator=cos
  Create 3x3 Matrix : sharedutil/Create 3x3 Matrix  aMode=aMode
      settings: LibrarySourceBlock=aerolibutil/Create 3x3 Matrix
  Demux : Demux  Outputs=3
  Divide : Product  Inputs=*/
  Divide1 : Product  Inputs=*/
  Matrix Multiply : Product  Multiplication=Matrix(*)
  Product2 : Product
  Product3 : Product
  Sin : Trigonometry
  Tan : Trigonometry  Operator=tan
  Terminator : Terminator
  Unary Minus : UnaryMinus
  eulerdot : Outport
  wires:
  omega/1 -> Matrix Multiply/2
  Matrix Multiply/1 -> eulerdot/1
  euler/1 -> Demux/1
  Demux/1 -> Sin/1, Cos/1  "phi"
  Demux/2 -> Tan/1, Cos1/1  "theta"
  Demux/3 -> Terminator/1  "psi"
  Constant/1 -> Create 3x3 Matrix/1
  Constant1/1 -> Create 3x3 Matrix/4, Create 3x3 Matrix/7
  Cos/1 -> Create 3x3 Matrix/5, Product2/1, Divide/1
  Sin/1 -> Product3/1, Unary Minus/1, Divide1/1
  Unary Minus/1 -> Create 3x3 Matrix/6
  Divide/1 -> Create 3x3 Matrix/9
  Divide1/1 -> Create 3x3 Matrix/8
  Product2/1 -> Create 3x3 Matrix/3
  Product3/1 -> Create 3x3 Matrix/2
  Tan/1 -> Product2/2, Product3/2
  Cos1/1 -> Divide1/2, Divide/2
  Create 3x3 Matrix/1 -> Matrix Multiply/1

== system RCAM_sim/RCAM/Aerodynamics/CLWingBody/If Action Subsystem ==
  alpha : Inport
  Action Port : ActionPort  ActionPortLabel=else
  Polynomial : Polyval  Coefs=[a3 a2 a1 a0]
  Out1 : Outport
  wires:
  Polynomial/1 -> Out1/1
  alpha/1 -> Polynomial/1

== system RCAM_sim/RCAM/Aerodynamics/CLWingBody/If Action Subsystem1 ==
  alpha : Inport
  Action Port : ActionPort  ActionPortLabel=if(u1 >= u2)
  Constant : Constant  Value=alpha_L0
  Gain : Gain  Gain=n
  Sum : Sum  Inputs=|+-
  CL_wb : Outport
  wires:
  alpha/1 -> Sum/1
  Constant/1 -> Sum/2
  Sum/1 -> Gain/1
  Gain/1 -> CL_wb/1
